simulink model "Single_phase_Half_wave_rectifiers"  (R2025b)
settings: Solver=ode23tb  StartTime=0.0  StopTime=0.1  RelTol=1e-3
libraries: spsVoltageMeasurementLib x4, spsACVoltageSourceLib x2, spsSeriesRLCBranchLib x2, spsDiodeLib x1, spsThyristorLib x1, sps_lib x1
settings Model: Creator=Luqmaan  LastModifiedBy=Luqmaan

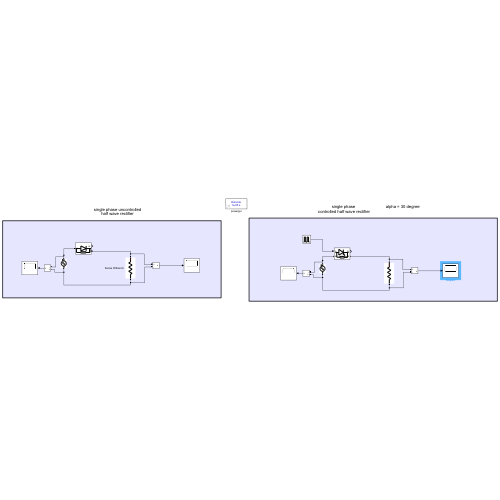
[thumbnail: Simulink's stored preview of the top-level diagram]
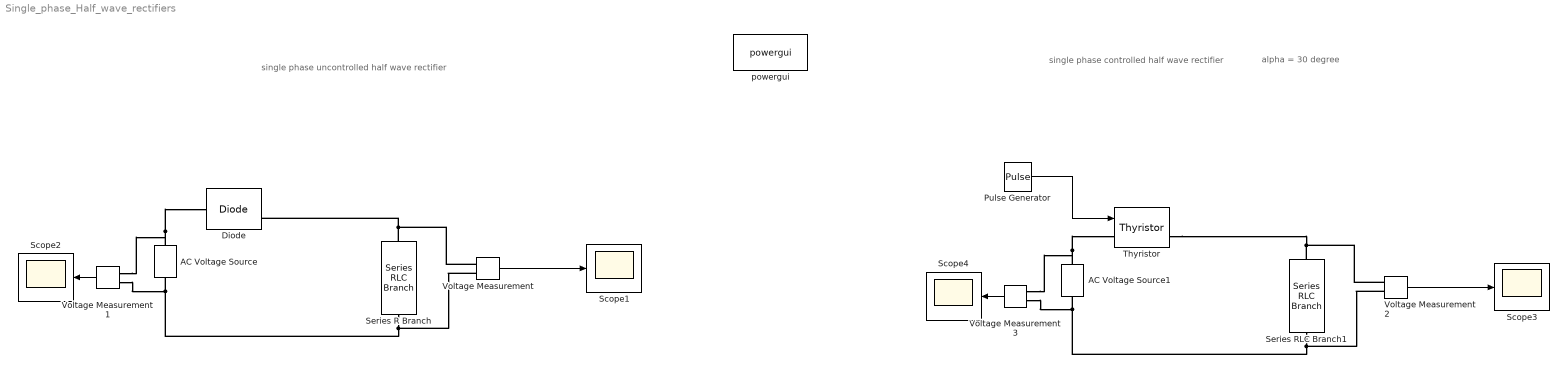
== system Single_phase_Half_wave_rectifiers ==
  note: single phase uncontrolled half wave rectifier
  note: single phase
      | controlled half wave rectifier
  note: alpha = 30 degree
  AC Voltage Source : spsACVoltageSourceLib/AC Voltage Source  Amplitude=325  Phase=0  Frequency=50  SampleTime=0  Measurements=None  BusType=swing  Pref=10e3  Qref=0  Qmin=-inf  Qmax=+inf
  AC Voltage Source1 : spsACVoltageSourceLib/AC Voltage Source  Amplitude=325  Phase=0  Frequency=50  SampleTime=0  Measurements=None  BusType=swing  Pref=10e3  Qref=0  Qmin=-inf  Qmax=+inf
  Diode : spsDiodeLib/Diode  Ron=0.001  Lon=0  Vf=0.8  IC=0  UseSnubber=0  Rs=500  Cs=250e-9  Measurements=on
  Pulse Generator : DiscretePulseGenerator  PulseType=Time based  Period=0.02  PulseWidth=10  PhaseDelay=60*(0.02 / 360)  VectorParams1D=off
  Scope{1..4} (4 alike) : Scope
      Scope1 settings: ActiveDisplayYMinimum=-43.324847042482133  ActiveDisplayYMaximum=365.032491929642
      Scope2 settings: ActiveDisplayYMinimum=-1462.7109255648625  ActiveDisplayYMaximum=1007.733628166422  DataLoggingVariableName=ScopeData2
      Scope3 settings: ActiveDisplayYMinimum=2.9421341555855918  ActiveDisplayYMaximum=322.90079450967505
      Scope4 settings: ActiveDisplayYMinimum=-824.45371223502468  ActiveDisplayYMaximum=619.96405316804351  DataLoggingVariableName=ScopeData3
  Series R Branch : spsSeriesRLCBranchLib/Series RLC Branch  LConnTagsString=__new0  RConnTagsString=__new0  BranchType=R  Resistance=100  Inductance=0  SetiL0=off  InitialCurrent=0  Capacitance=inf  Setx0=off  InitialVoltage=0  Measurements=None
  Series RLC Branch1 : spsSeriesRLCBranchLib/Series RLC Branch  LConnTagsString=__new0  RConnTagsString=__new0  BranchType=R  Resistance=100  Inductance=0  SetiL0=off  InitialCurrent=0  Capacitance=inf  Setx0=off  InitialVoltage=0  Measurements=None
  Thyristor : spsThyristorLib/Thyristor  Ron=0.001  Lon=0  Vf=0.8  IC=0  Rs=500  Cs=250e-9  Measurements=on
  Voltage Measurement{,1..3} (4 alike) : spsVoltageMeasurementLib/Voltage Measurement  PhasorSimulation=off  OutputType=Complex  PSBequivalent=0
  powergui : sps_lib/powergui  Priority=1  SimulationMode=Discrete  SampleTime=1e-5  frequency=60  Iterations=50  frequencyindice=50  Pbase=100e6  ErrMax=1e-4  UnitsV=kV  UnitsW=MW  buscounter=0  FunctionMessages=off  echomessages=off  EnableUseOfTLC=off  CurrentSourceSwitches=off  DisableSnubberDevices=off  DisableRonSwitches=off  DisableVfSwitches=off  DisplayEquations=off  AutomaticDiscreteSolvers=off  SolverType=Tustin/Backward Euler (TBE)  Interpol=off  ExternalGateDelay=off  methode=off  Ts=100  x0status=blocks  SPID=on  SwTol=0  HookPort=off  NonlinearTolerance=1e-4  nMaxIteration=100  ContinueOnMaxIteration=off  RestoreLinks=warning  ResistiveCurrentMeasurement=off  Frange=[0:2:500]  Ylog=off  Xlog=on  ShowGrid=off  save=off  variable=ZData  structure=0  ZoomFFT=off  StartTime=0.0  cycles=1  DisplayStyle=1  fundamental=60  FreqAxis=off  MaxFrequency=1000  frequencyindicesteady=1  RmsSteady=1  display=off
  wires:
  Voltage Measurement/1 -> Scope1/1
  Voltage Measurement1/1 -> Scope2/1
  Voltage Measurement2/1 -> Scope3/1
  Voltage Measurement3/1 -> Scope4/1
  Pulse Generator/1 -> Thyristor/1
  connections:
  AC Voltage Source/RConn1 -- Voltage Measurement1/LConn2 -- Diode/LConn1
  Series R Branch/LConn1 -- Diode/RConn1 -- Voltage Measurement/LConn1
  Series R Branch/RConn1 -- Voltage Measurement/LConn2 -- Voltage Measurement1/LConn1 -- AC Voltage Source/LConn1
  Series RLC Branch1/LConn1 -- Thyristor/RConn1 -- Voltage Measurement2/LConn1
  Series RLC Branch1/RConn1 -- Voltage Measurement2/LConn2 -- Voltage Measurement3/LConn1 -- AC Voltage Source1/LConn1
  AC Voltage Source1/RConn1 -- Voltage Measurement3/LConn2 -- Thyristor/LConn1
